simulink model "vehicleCtl"  (R2016b)
settings: Solver=FixedStepAuto  StartTime=0.0  StopTime=300  FixedStep=0.1  RelTol=1e-3
model workspace (MAT data in the model file):
  Ffun : class16 (value not decoded)
  Fnominal = 156.500401939
  Gfun : class16 (value not decoded)
  Ki = 0.02
  Kt = 0
  TmaxAW = inf
  TminAW = -inf
  Tnominal = 0.210633111627
  myController = tf
  myController.IOSize_ = [1 1]
  myController.Data_ = ltipack.tfdata
  myController.Data_.num = {[0.2 0.45]}
  myController.Data_.den = {[0.15 1]}
  myController.Data_.Delay.Input = 0
  myController.Data_.Delay.Output = 0
  myController.Data_.Delay.IO = 0
  myController.Data_.Ts = 0
  tau = 0.1
  velocityRef = timeseries
  velocityRef.Name = 'unnamed'
  velocityRef.DataInfo = tsdata.datametadata
  velocityRef.DataInfo.Interpolation = tsdata.interpolation
  velocityRef.DataInfo.Interpolation.Fhandle : function handle (value not decoded)
  velocityRef.DataInfo.Interpolation.Name = 'linear'
  velocityRef.TimeInfo = tsdata.timemetadata
  velocityRef.TimeInfo.Length = 3001
  velocityRef.TimeInfo.DuplicateTimes = 0
  velocityRef.TimeInfo.Time_ = [0 0.1 0.2 0.3 0.4 0.5 0.6 0.7 0.8 0.9 1 1.1 ... (3001 elements, 3001x1)]
  velocityRef.TimeInfo.Initialized = 1
  velocityRef.QualityInfo = tsdata.qualmetadata
  velocityRef.Data_ = [90.0720868889 90.0720868889 90.0720868889 90.0720868889 90.0720868889 90.0720868889 90.0720868889 90.0720868889 90.0720868889 90.0720868889 90.0720868889 90.0720868889 ... (3001 elements, 3001x1)]
  vnominal = 90.0720868889
  vnominalms = 25.0200241358
symbols that are objects in the model workspace (value not decoded): Ffun, Gfun
libraries: cstblocks x1
settings Model: Creator=jamessaunderson  LastModifiedBy=jsau0001
settings DataIOCC: ReturnWorkspaceOutputs=on
settings SFSimCC: SimUseLocalCustomCode=on
settings RTWCC: RTWUseLocalCustomCode=on

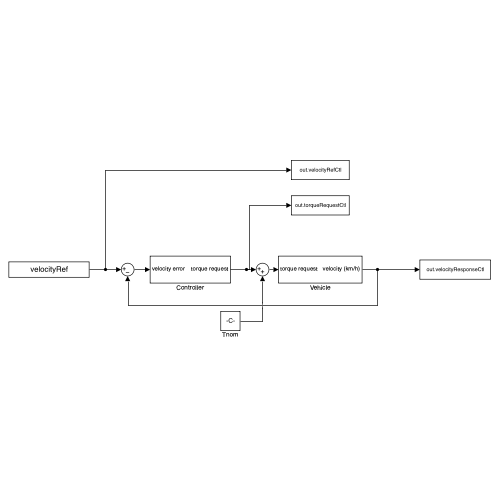
[thumbnail: Simulink's stored preview of the top-level diagram]
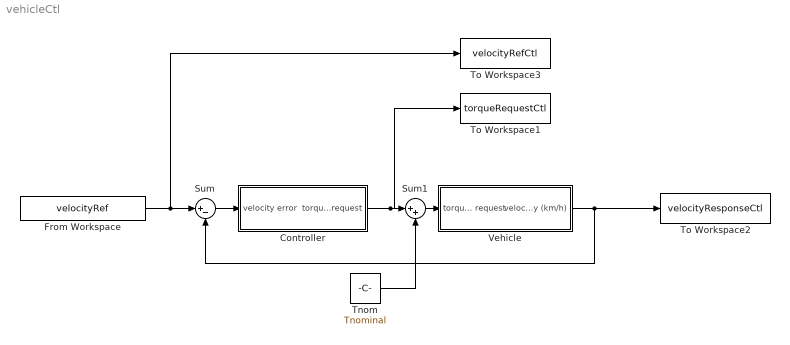
== system vehicleCtl ==
  Controller : Subsystem
  From Workspace : FromWorkspace  VariableName=velocityRef  OutputAfterFinalValue=Holding final value
  Sum : Sum  Inputs=|+-
  Sum1 : Sum  Inputs=|++
  Tnom : Constant  Value=Tnominal
  To Workspace1 : ToWorkspace  VariableName=torqueRequestCtl  SaveFormat=Timeseries  SampleTime=-1
  To Workspace2 : ToWorkspace  VariableName=velocityResponseCtl  SaveFormat=Timeseries  SampleTime=-1
  To Workspace3 : ToWorkspace  VariableName=velocityRefCtl  SaveFormat=Timeseries  SampleTime=-1
  Vehicle : Subsystem
  wires:
  Vehicle/1(velocity (km/h)) -> Sum/2, To Workspace2/1
  Controller/1(torque request) -> To Workspace1/1, Sum1/1
  From Workspace/1 -> To Workspace3/1, Sum/1
  Sum/1 -> Controller/1(velocity error)
  Sum1/1 -> Vehicle/1(torque request)
  Tnom/1 -> Sum1/2

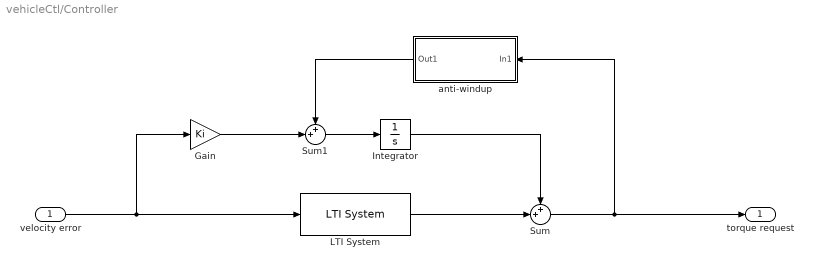
== system vehicleCtl/Controller ==
  velocity error : Inport
  Gain : Gain  Gain=Ki
  Integrator : Integrator
  LTI System : cstblocks/LTI System  sys=myController  IC=[]
  Sum : Sum  Inputs=++|
  Sum1 : Sum  Inputs=++|
  anti-windup : Subsystem
  torque request : Outport
  wires:
  velocity error/1 -> Gain/1, LTI System/1
  Sum/1 -> torque request/1, anti-windup/1(In1)
  Gain/1 -> Sum1/2
  Sum1/1 -> Integrator/1
  anti-windup/1(Out1) -> Sum1/1
  LTI System/1 -> Sum/2
  Integrator/1 -> Sum/1

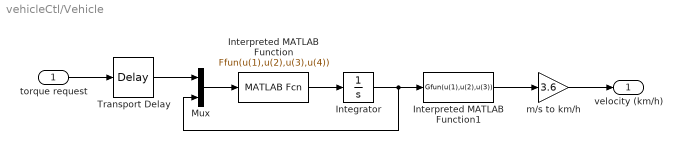
== system vehicleCtl/Vehicle ==
  torque request : Inport
  Integrator : Integrator  InitialCondition=[0;vnominalms;Fnominal]
  Interpreted MATLAB Function : MATLABFcn  MATLABFcn=Ffun(u(1),u(2),u(3),u(4))  OutputDimensions=3
  Interpreted MATLAB Function1 : MATLABFcn  MATLABFcn=Gfun(u(1),u(2),u(3))  OutputDimensions=1
  Mux : Mux  Inputs=2
  Transport Delay : TransportDelay  DelayTime=tau  InitialOutput=Tnominal
  m/s to km/h : Gain  Gain=3.6
  velocity (km/h) : Outport
  wires:
  Transport Delay/1 -> Mux/1
  torque request/1 -> Transport Delay/1
  Interpreted MATLAB Function/1 -> Integrator/1
  Integrator/1 -> Mux/2, Interpreted MATLAB Function1/1
  Mux/1 -> Interpreted MATLAB Function/1
  Interpreted MATLAB Function1/1 -> m/s to km/h/1
  m/s to km/h/1 -> velocity (km/h)/1

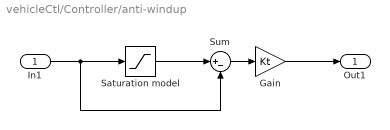
== system vehicleCtl/Controller/anti-windup ==
  In1 : Inport
  Gain : Gain  Gain=Kt
  Saturation model : Saturate  UpperLimit=TmaxAW  LowerLimit=TminAW
  Sum : Sum  Inputs=|+-
  Out1 : Outport
  wires:
  Saturation model/1 -> Sum/1
  In1/1 -> Sum/2, Saturation model/1
  Sum/1 -> Gain/1
  Gain/1 -> Out1/1
